simulink model "Minh_Final_project_Inverter_V3"  (R2024b)
settings: Solver=VariableStepAuto  StartTime=0.0  StopTime=100  FixedStep=1e-5  MaxStep=1e-3  MinStep=1e-8  RelTol=1e-2
values from neighbouring files (symbols this model uses):
  A_f = 1.24    [Minh_Inverter_Init.m]
  C_d = 0.7041    [Minh_Inverter_Init.m]
  C_rr = 0.02    [Minh_Inverter_Init.m]
  Current_max = min(InvCurr,mCurr)    [Minh_Inverter_Init.m]
  Encoder_Offset = (PhaseA_offset/ppair)*pi/180    (= -0.785398163397)    [Minh_Inverter_Init.m]
  g = 9.8    [Minh_Inverter_Init.m]
  J = mrot*r^2/k^2 + 0.0045    (= 0.8303048)    [Minh_Inverter_Init.m]
  k = 1    [Minh_Inverter_Init.m]
  lambda = 0.0375    [Minh_Inverter_Init.m]
  Ld = 0.1e-3    (= 0.0001)    [Minh_Inverter_Init.m]
  Lq = Ld    (= 0.0001)    [Minh_Inverter_Init.m]
  m = 1    [Minh_Inverter_Init.m]
  ppair = 4    [Minh_Inverter_Init.m]
  r = 0.4064/2    (= 0.2032)    [Minh_Inverter_Init.m]
  rho = 1.2    [Minh_Inverter_Init.m]
  Rs = (Rpp^2)/(Rpp*3)    (= 0.00433333333333)    [Minh_Inverter_Init.m]
  speed_max = rpm_max*2*pi/60    (= 523.598775598)    [Minh_Inverter_Init.m]
  Torque_max = Current_max*3*lambda*ppair/2    [Minh_Inverter_Init.m]
  Voltage_max = min(V_bat,mVolt)    [Minh_Inverter_Init.m]
undefined symbols (not defined in the file or in its folder): Down, Up
libraries: nesl_utility x27, fl_lib x23, slpidlib x12, ee_lib x11, spsabctodq0Lib x4, simulink x3, spsdq0toabcLib x2, eePwmGenerator x2, mcbresolverdecoderlib x1, eeResolverToDigitalConverter x1
(part 1 of 3)
settings Model: ExtModeTrigDuration=8  Creator=minhp  LastModifiedBy=minhp
settings SolverCC: ZeroCrossControl=DisableAll  ZeroCrossAlgorithm=Adaptive
settings OptimizationCC: DefaultParameterBehavior=Inlined  UseDivisionForNetSlopeComputation=on  GainParamInheritBuiltInType=on  UseFloatMulNetSlope=on  DefaultUnderspecifiedDataType=single  InlineInvariantSignals=on  PassReuseOutputArgsAs=Individual arguments  ZeroExternalMemoryAtStartup=off  NoFixptDivByZeroProtection=on  EfficientFloat2IntCast=on  LifeSpan=1  MaxStackSize=1024  OptimizeBlockOrder=speed  DifferentSizesBufferReuse=on  EfficientTunableParamExpr=on
settings DebuggingCC: MaskedZcDiagnostic=none  IgnoredZcDiagnostic=none  ParameterTunabilityLossMsg=error
settings HardwareCC: ProdBitPerChar=16  ProdBitPerInt=16  ProdBitPerPointer=32  ProdBitPerSizeT=32  ProdBitPerPtrDiffT=32  ProdLargestAtomicInteger=Integer  ProdLargestAtomicFloat=None  ProdWordSize=16  ProdLongLongMode=on  ProdHWDeviceType=Texas Instruments->C2000  HardwareBoardFeatureSet=SoCBlockset
settings SFSimCC: MATLABDynamicMemAlloc=off
settings RTWCC: Description=Embedded Coder  SystemTargetFile=ert.tlc  HardwareBoard=TI Piccolo F280049C LaunchPad  GenCodeOnly=on  TemplateMakefile=ert_default_tmf  Toolchain=Texas Instruments Code Composer Studio (C2000)  CodeProfilingSaveOptions=MetricsOnly
settings CodeAppCC: ForceParamTrailComments=on  IgnoreCustomStorageClasses=off  OperatorAnnotations=on  SimulinkDataObjDesc=on  SFDataObjDesc=on  CustomSymbolStrGlobalVar=rt$N$M  CustomSymbolStrType=$N$M  CustomSymbolStrFcn=$N$M$F  CustomSymbolStrMacro=$N$M  InsertBlockDesc=on
settings ERTTargetCC: CodeReplacementLibrary=TI C28x  IncludeMdlTerminateFcn=off  CombineSignalStateStructs=on  SupportAbsoluteTime=off  SupportComplex=off  SupportContinuousTime=on  ExtModeTransport=4  ExtModeStaticAlloc=on  ExtModeAutomaticAllocSize=off  ExtModeStaticAllocSize=5000  ExtModeMexFile=ext_xcp  ExtModeIntrfLevel=Level2 - Open  ERTFilePackagingFormat=CompactWithDataFile  DynamicArrayContainerType=coder::array

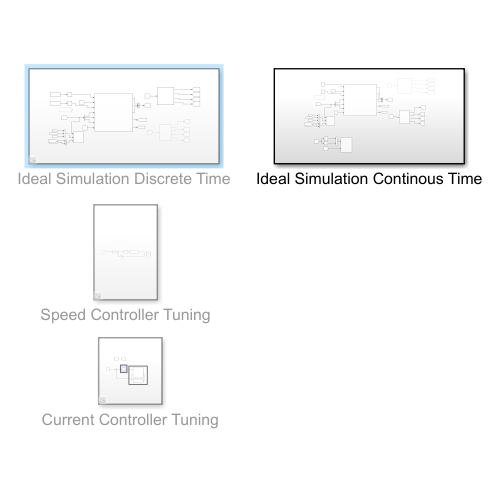
[thumbnail: Simulink's stored preview of the top-level diagram]
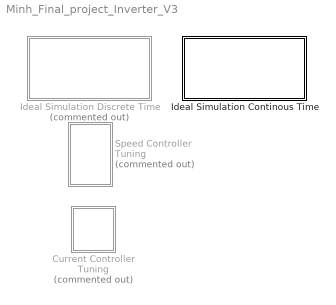
== system Minh_Final_project_Inverter_V3 ==
  Current Controller Tuning : Subsystem  Commented=on
  Ideal Simulation Continous Time : Subsystem
  Ideal Simulation Discrete Time : Subsystem  Commented=on
  Speed Controller Tuning : Subsystem  Commented=on

== system Minh_Final_project_Inverter_V3/Current Controller Tuning ==
  note: Use the PID tuner app to tune for bandwidth of at least 2000rad/s
      | and PM of 90deg
  note: Q current
      | Cntrl
  note: PMSM (Mathematical Model)
  I_dq PID : slpidlib/PID Controller  Controller=PI  Form=Parallel  TimeDomain=Continuous-time  UseExternalTs=off  SampleTime=-1  IntegratorMethod=Forward Euler  FilterMethod=Forward Euler  ControllerParametersSource=internal  P=0.199995991549269  I=7.0005743607815  UseKiTs=off  D=2.81416629288768e-05  UseExternalDerivativeSource=off  N=4271.19819316481  UseFilter=on  TunerSelectOption=Transfer Function Based (PID Tuner App)  InitialConditionSource=internal  InitialConditionForIntegrator=0  InitialConditionForFilter=0  DifferentiatorICPrevScaledInput=0  ExternalReset=none  TrackingMode=off  Kt=1  LimitOutput=on  SatLimitsSource=internal  UpperSaturationLimit=Voltage_max  LowerSaturationLimit=-Voltage_max  LinearizeAsGain=off  AntiWindupMode=none  Kb=1  LimitIntegrator=on  UpperIntegratorSaturationLimit=Voltage_max  LowerIntegratorSaturationLimit=-Voltage_max  POutMin=[]  POutMax=[]  IOutMin=[]  IOutMax=[]  DOutMin=[]  DOutMax=[]  NOutMin=[]  NOutMax=[]  SumOutMin=[]  SumOutMax=[]  SaturationOutMin=[]  SaturationOutMax=[]  PParamMin=[]  PParamMax=[]  IParamMin=[]  IParamMax=[]  DParamMin=[]  DParamMax=[]  NParamMin=[]  NParamMax=[]  KbParamMin=[]  KbParamMax=[]  KtParamMin=[]  KtParamMax=[]  KbOutMin=[]  KbOutMax=[]  KtOutMin=[]  KtOutMax=[]  IntegratorOutMin=[]  IntegratorOutMax=[]  FilterOutMin=[]  FilterOutMax=[]  SumI1OutMin=[]  SumI1OutMax=[]  SumI2OutMin=[]  SumI2OutMax=[]  SumI3OutMin=[]  SumI3OutMax=[]  SumI4OutMin=[]  SumI4OutMax=[]  SumDOutMin=[]  SumDOutMax=[]  DifferentiatorOutMin=[]  DifferentiatorOutMax=[]  FilterDiffOutCoefMin=[]  FilterDiffOutCoefMax=[]  ReciprocalOutMin=[]  ReciprocalOutMax=[]  SumDenOutMin=[]  SumDenOutMax=[]  SumNumOutMin=[]  SumNumOutMax=[]  DivideOutMin=[]  DivideOutMax=[]  UdiffTsProdOutMin=[]  UdiffTsProdOutMax=[]  NTsProdOutMin=[]  NTsProdOutMax=[]  UintegralTsProdOutMin=[]  UintegralTsProdOutMax=[]  UngainTsProdOutMin=[]  UngainTsProdOutMax=[]  ClampingZeroOutDataTypeStr=Inherit: Inherit via back propagation  ClampingZeroOutMin=[]  ClampingZeroOutMax=[]  FilterDenConstantOutDataTypeStr=Inherit: Inherit via back propagation  FilterDenConstantOutMin=[]  FilterDenConstantOutMax=[]  PCopyOutDataTypeStr=Inherit: Inherit via back propagation  PCopyOutMin=[]  PCopyOutMax=[]  NCopyOutDataTypeStr=Inherit: Inherit via back propagation  NCopyOutMin=[]  NCopyOutMax=[]  IntegratorContinuousStateAttributes=''  IntegratorStateMustResolveToSignalObject=off  IntegratorRTWStateStorageClass=Auto  FilterContinuousStateAttributes=''  FilterStateMustResolveToSignalObject=off  FilterRTWStateStorageClass=Auto  ParallelPVariant=InternalParameters  IdealPVariant=Disabled  IVariant=InternalParameters  DVariant=Disabled  IntegratorVariant=Continuous  SatVariant=Enabled  AWVariant=Passthrough  PCopyVariant=Disabled  TRVariant=Disabled  FdbkBlocksVariant=Forward  IdealPFdbkVariant=Disabled  SatFdbkVariant=Disabled  DerivativeFilterVariant=Disabled  NVariant=Disabled  NCopyVariant=Disabled_SignalSpec  FilterICVariant=Disabled  IntegratorICVariant=InternalICs  ExternalResetVariant=Disabled  TRSumVariant=Passthrough  SumFdbkVariant=Disabled  SumVariant=Sum_PI  TsampFilterVariant=InternalTs  TsampNgainVariant=Passthrough  TsampIntegralVariant=Disabled_SignalSpec  ExternalSaturationOutDataTypeStr=Inherit: Same as second input  DerivativeSourceVariant=Disabled  PreIntVariant=InternalPreInt
  I_dq PID1 : slpidlib/PID Controller  Commented=on  Controller=PID  Form=Parallel  TimeDomain=Discrete-time  UseExternalTs=off  SampleTime=-1  IntegratorMethod=Forward Euler  FilterMethod=Forward Euler  ControllerParametersSource=internal  P=0.183534072898089  I=62.295633089485  UseKiTs=off  D=2.81416629288768e-05  UseExternalDerivativeSource=off  N=4271.19819316481  UseFilter=on  TunerSelectOption=Transfer Function Based (PID Tuner App)  InitialConditionSource=internal  InitialConditionForIntegrator=0  InitialConditionForFilter=0  DifferentiatorICPrevScaledInput=0  ExternalReset=none  TrackingMode=off  Kt=1  LimitOutput=on  SatLimitsSource=internal  UpperSaturationLimit=Voltage_max  LowerSaturationLimit=-Voltage_max  LinearizeAsGain=off  AntiWindupMode=none  Kb=1  LimitIntegrator=on  UpperIntegratorSaturationLimit=Voltage_max  LowerIntegratorSaturationLimit=-Voltage_max  POutMin=[]  POutMax=[]  IOutMin=[]  IOutMax=[]  DOutMin=[]  DOutMax=[]  NOutMin=[]  NOutMax=[]  SumOutMin=[]  SumOutMax=[]  SaturationOutMin=[]  SaturationOutMax=[]  PParamMin=[]  PParamMax=[]  IParamMin=[]  IParamMax=[]  DParamMin=[]  DParamMax=[]  NParamMin=[]  NParamMax=[]  KbParamMin=[]  KbParamMax=[]  KtParamMin=[]  KtParamMax=[]  KbOutMin=[]  KbOutMax=[]  KtOutMin=[]  KtOutMax=[]  IntegratorOutMin=[]  IntegratorOutMax=[]  FilterOutMin=[]  FilterOutMax=[]  SumI1OutMin=[]  SumI1OutMax=[]  SumI2OutMin=[]  SumI2OutMax=[]  SumI3OutMin=[]  SumI3OutMax=[]  SumI4OutMin=[]  SumI4OutMax=[]  SumDOutMin=[]  SumDOutMax=[]  DifferentiatorOutMin=[]  DifferentiatorOutMax=[]  FilterDiffOutCoefMin=[]  FilterDiffOutCoefMax=[]  ReciprocalOutMin=[]  ReciprocalOutMax=[]  SumDenOutMin=[]  SumDenOutMax=[]  SumNumOutMin=[]  SumNumOutMax=[]  DivideOutMin=[]  DivideOutMax=[]  UdiffTsProdOutMin=[]  UdiffTsProdOutMax=[]  NTsProdOutMin=[]  NTsProdOutMax=[]  UintegralTsProdOutMin=[]  UintegralTsProdOutMax=[]  UngainTsProdOutMin=[]  UngainTsProdOutMax=[]  ClampingZeroOutDataTypeStr=Inherit: Inherit via back propagation  ClampingZeroOutMin=[]  ClampingZeroOutMax=[]  FilterDenConstantOutDataTypeStr=Inherit: Inherit via back propagation  FilterDenConstantOutMin=[]  FilterDenConstantOutMax=[]  PCopyOutDataTypeStr=Inherit: Inherit via back propagation  PCopyOutMin=[]  PCopyOutMax=[]  NCopyOutDataTypeStr=Inherit: Inherit via back propagation  NCopyOutMin=[]  NCopyOutMax=[]  IntegratorContinuousStateAttributes=''  IntegratorStateMustResolveToSignalObject=off  IntegratorRTWStateStorageClass=Auto  FilterContinuousStateAttributes=''  FilterStateMustResolveToSignalObject=off  FilterRTWStateStorageClass=Auto  ParallelPVariant=InternalParameters  IdealPVariant=Disabled  IVariant=InternalParameters  DVariant=InternalParameters  IntegratorVariant=Discrete  SatVariant=Enabled  AWVariant=Passthrough  PCopyVariant=Disabled  TRVariant=Disabled  FdbkBlocksVariant=Forward  IdealPFdbkVariant=Disabled  SatFdbkVariant=Disabled  DerivativeFilterVariant=ForwardEulerFilter  NVariant=InternalParameters  NCopyVariant=Disabled  FilterICVariant=InternalICsFilter  IntegratorICVariant=InternalICs  ExternalResetVariant=Disabled  TRSumVariant=Passthrough  SumFdbkVariant=Disabled  SumVariant=Sum_PID  TsampFilterVariant=InternalTs  TsampNgainVariant=Passthrough  TsampIntegralVariant=Disabled_SignalSpec  ExternalSaturationOutDataTypeStr=Inherit: Same as second input  DerivativeSourceVariant=ErrorSignal  PreIntVariant=InternalPreInt
  I_dq PID2 : slpidlib/PID Controller  Commented=on  Controller=PI  Form=Parallel  TimeDomain=Discrete-time  UseExternalTs=off  SampleTime=-1  IntegratorMethod=Forward Euler  FilterMethod=Forward Euler  ControllerParametersSource=internal  P=0.216674080570424  I=8.23559930371868  UseKiTs=off  D=2.81416629288768e-05  UseExternalDerivativeSource=off  N=4271.19819316481  UseFilter=on  TunerSelectOption=Transfer Function Based (PID Tuner App)  InitialConditionSource=internal  InitialConditionForIntegrator=0  InitialConditionForFilter=0  DifferentiatorICPrevScaledInput=0  ExternalReset=none  TrackingMode=off  Kt=1  LimitOutput=on  SatLimitsSource=internal  UpperSaturationLimit=Voltage_max  LowerSaturationLimit=-Voltage_max  LinearizeAsGain=off  AntiWindupMode=none  Kb=1  LimitIntegrator=on  UpperIntegratorSaturationLimit=Voltage_max  LowerIntegratorSaturationLimit=-Voltage_max  POutMin=[]  POutMax=[]  IOutMin=[]  IOutMax=[]  DOutMin=[]  DOutMax=[]  NOutMin=[]  NOutMax=[]  SumOutMin=[]  SumOutMax=[]  SaturationOutMin=[]  SaturationOutMax=[]  PParamMin=[]  PParamMax=[]  IParamMin=[]  IParamMax=[]  DParamMin=[]  DParamMax=[]  NParamMin=[]  NParamMax=[]  KbParamMin=[]  KbParamMax=[]  KtParamMin=[]  KtParamMax=[]  KbOutMin=[]  KbOutMax=[]  KtOutMin=[]  KtOutMax=[]  IntegratorOutMin=[]  IntegratorOutMax=[]  FilterOutMin=[]  FilterOutMax=[]  SumI1OutMin=[]  SumI1OutMax=[]  SumI2OutMin=[]  SumI2OutMax=[]  SumI3OutMin=[]  SumI3OutMax=[]  SumI4OutMin=[]  SumI4OutMax=[]  SumDOutMin=[]  SumDOutMax=[]  DifferentiatorOutMin=[]  DifferentiatorOutMax=[]  FilterDiffOutCoefMin=[]  FilterDiffOutCoefMax=[]  ReciprocalOutMin=[]  ReciprocalOutMax=[]  SumDenOutMin=[]  SumDenOutMax=[]  SumNumOutMin=[]  SumNumOutMax=[]  DivideOutMin=[]  DivideOutMax=[]  UdiffTsProdOutMin=[]  UdiffTsProdOutMax=[]  NTsProdOutMin=[]  NTsProdOutMax=[]  UintegralTsProdOutMin=[]  UintegralTsProdOutMax=[]  UngainTsProdOutMin=[]  UngainTsProdOutMax=[]  ClampingZeroOutDataTypeStr=Inherit: Inherit via back propagation  ClampingZeroOutMin=[]  ClampingZeroOutMax=[]  FilterDenConstantOutDataTypeStr=Inherit: Inherit via back propagation  FilterDenConstantOutMin=[]  FilterDenConstantOutMax=[]  PCopyOutDataTypeStr=Inherit: Inherit via back propagation  PCopyOutMin=[]  PCopyOutMax=[]  NCopyOutDataTypeStr=Inherit: Inherit via back propagation  NCopyOutMin=[]  NCopyOutMax=[]  IntegratorContinuousStateAttributes=''  IntegratorStateMustResolveToSignalObject=off  IntegratorRTWStateStorageClass=Auto  FilterContinuousStateAttributes=''  FilterStateMustResolveToSignalObject=off  FilterRTWStateStorageClass=Auto  ParallelPVariant=InternalParameters  IdealPVariant=Disabled  IVariant=InternalParameters  DVariant=Disabled  IntegratorVariant=Discrete  SatVariant=Enabled  AWVariant=Passthrough  PCopyVariant=Disabled  TRVariant=Disabled  FdbkBlocksVariant=Forward  IdealPFdbkVariant=Disabled  SatFdbkVariant=Disabled  DerivativeFilterVariant=Disabled  NVariant=Disabled  NCopyVariant=Disabled_SignalSpec  FilterICVariant=Disabled  IntegratorICVariant=InternalICs  ExternalResetVariant=Disabled  TRSumVariant=Passthrough  SumFdbkVariant=Disabled  SumVariant=Sum_PI  TsampFilterVariant=InternalTs  TsampNgainVariant=Passthrough  TsampIntegralVariant=Disabled_SignalSpec  ExternalSaturationOutDataTypeStr=Inherit: Same as second input  DerivativeSourceVariant=Disabled  PreIntVariant=InternalPreInt
  Machine Model in DQ1 : Subsystem
  Mechanical Model : Subsystem
  Sum3 : Sum  Inputs=|+-
  current request1 : Constant  Value=10
  wires:
  Machine Model in DQ1/1(i_q) -> Sum3/2  "i_q"
  Machine Model in DQ1/2(T_e) -> Mechanical Model/1(T_e)  "Tourqe"
  current request1/1 -> Sum3/1
  Sum3/1 -> I_dq PID/1  "Iq_error"
  I_dq PID/1 -> Machine Model in DQ1/1(v_q)  "Vq*"
  Mechanical Model/1(w_m) -> Machine Model in DQ1/2(w_m)

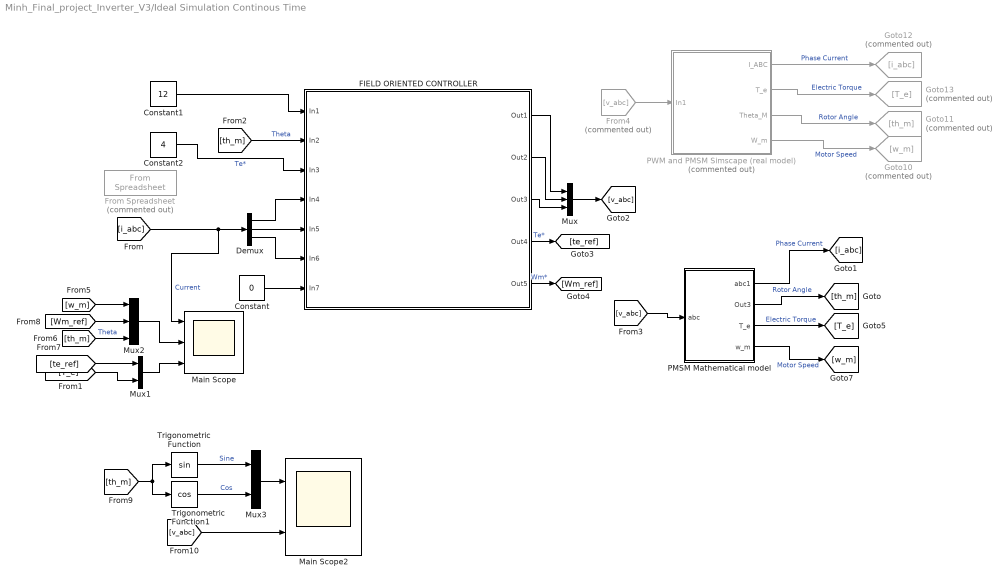
== system Minh_Final_project_Inverter_V3/Ideal Simulation Continous Time ==
  Constant : Constant  Value=0
  Constant1 : Constant  Value=12
  Constant2 : Constant  Value=4
  Demux : Demux  Outputs=3
  FIELD ORIENTED CONTROLLER : Subsystem
  From Spreadsheet : FromSpreadsheet  Commented=on  FileName=Inverter_Lap_Sim_Current_Calcs.xlsx
  From4 : From  Commented=on  GotoTag=v_abc
  Goto10 : Goto  Commented=on  GotoTag=w_m
  Goto11 : Goto  Commented=on  GotoTag=th_m
  Goto12 : Goto  Commented=on  GotoTag=i_abc
  Goto13 : Goto  Commented=on  GotoTag=T_e
  Main Scope : Scope  NumInputPorts=3
  Main Scope2 : Scope  NumInputPorts=2
  Mux : Mux  Inputs=3
  Mux1 : Mux  Inputs=2
  Mux2 : Mux  Inputs=3
  Mux3 : Mux  Inputs=2
  PMSM Mathematical model : Subsystem
  PWM and PMSM Simscape (real model) : Subsystem  Commented=on
  Trigonometric Function : Trigonometry
  Trigonometric Function1 : Trigonometry  Operator=cos
  wires:
  [th_m] -> FIELD ORIENTED CONTROLLER/2(In2)  "Theta"
  FIELD ORIENTED CONTROLLER/3(Out3) -> Mux/3
  [i_abc] -> Main Scope/1, Demux/1  "Current"
  Mux2/1 -> Main Scope/2
  [te_ref] -> Mux1/1
  Constant/1 -> FIELD ORIENTED CONTROLLER/7(In7)
  PWM and PMSM Simscape (real model)/3(Theta_M) -> Goto11/1  "Rotor Angle"
  [T_e] -> Mux1/2
  FIELD ORIENTED CONTROLLER/2(Out2) -> Mux/2
  Demux/3 -> FIELD ORIENTED CONTROLLER/6(In6)
  FIELD ORIENTED CONTROLLER/5(Out5) -> [Wm_ref]  "Wm*"
  Demux/2 -> FIELD ORIENTED CONTROLLER/5(In5)
  PMSM Mathematical model/4(w_m) -> [w_m]  "Motor Speed"
  FIELD ORIENTED CONTROLLER/4(Out4) -> [te_ref]  "Te*"
  FIELD ORIENTED CONTROLLER/1(Out1) -> Mux/1
  PMSM Mathematical model/2(Out3) -> [th_m]  "Rotor Angle"
  Demux/1 -> FIELD ORIENTED CONTROLLER/4(In4)
  Mux/1 -> [v_abc]
  [th_m] -> Mux2/3  "Theta"
  [w_m] -> Mux2/1
  PWM and PMSM Simscape (real model)/2(T_e) -> Goto13/1  "Electric Torque"
  Constant2/1 -> FIELD ORIENTED CONTROLLER/3(In3)  "Te*"
  PWM and PMSM Simscape (real model)/1(I_ABC) -> Goto12/1  "Phase Current"
  From4/1 -> PWM and PMSM Simscape (real model)/1(In1)
  PWM and PMSM Simscape (real model)/4(W_m) -> Goto10/1  "Motor Speed"
  [v_abc] -> PMSM Mathematical model/1(abc)
  PMSM Mathematical model/1(abc1) -> [i_abc]  "Phase Current"
  PMSM Mathematical model/3(T_e) -> [T_e]  "Electric Torque"
  Constant1/1 -> FIELD ORIENTED CONTROLLER/1(In1)
  [Wm_ref] -> Mux2/2
  Mux1/1 -> Main Scope/3
  Trigonometric Function1/1 -> Mux3/2  "Cos"
  Mux3/1 -> Main Scope2/1
  [v_abc] -> Main Scope2/2
  Trigonometric Function/1 -> Mux3/1  "Sine"
  [th_m] -> Trigonometric Function1/1, Trigonometric Function/1

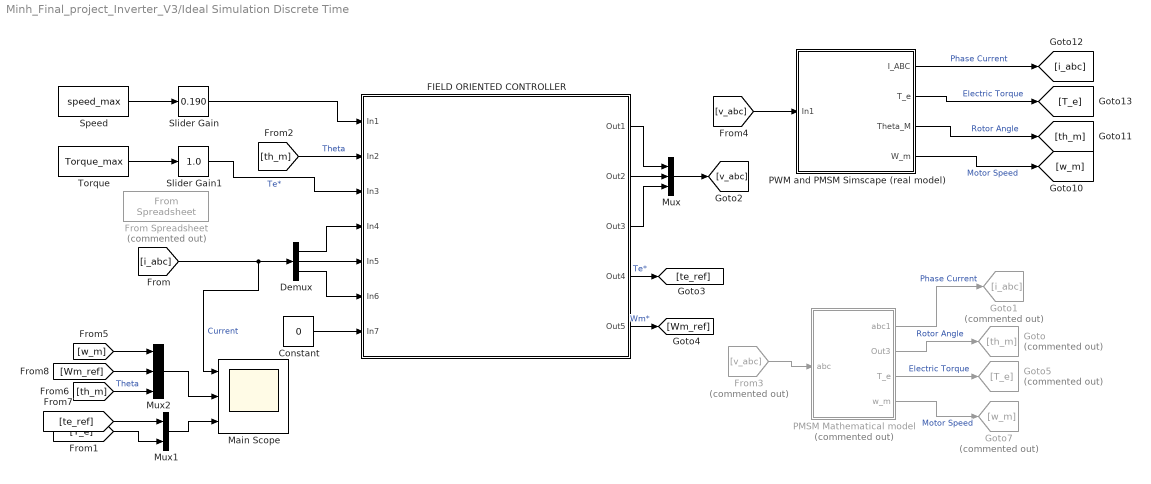
== system Minh_Final_project_Inverter_V3/Ideal Simulation Discrete Time ==
  Constant : Constant  Value=0
  Demux : Demux  Outputs=3
  FIELD ORIENTED CONTROLLER : Subsystem
  From Spreadsheet : FromSpreadsheet  Commented=on  FileName=Inverter_Lap_Sim_Current_Calcs.xlsx
  From3 : From  Commented=on  GotoTag=v_abc
  Goto : Goto  Commented=on  GotoTag=th_m
  Goto1 : Goto  Commented=on  GotoTag=i_abc
  Goto5 : Goto  Commented=on  GotoTag=T_e
  Goto7 : Goto  Commented=on  GotoTag=w_m
  Main Scope : Scope  NumInputPorts=3
  Mux : Mux  Inputs=3
  Mux1 : Mux  Inputs=2
  Mux2 : Mux  Inputs=3
  PMSM Mathematical model : Subsystem  Commented=on
  PWM and PMSM Simscape (real model) : Subsystem
  Slider Gain : simulink/Math Operations/Slider Gain  gain=0.190  low=0  high=1
  Slider Gain1 : simulink/Math Operations/Slider Gain  gain=1.0  low=0  high=1
  Speed : Constant  Value=speed_max
  Torque : Constant  Value=Torque_max
  wires:
  [th_m] -> FIELD ORIENTED CONTROLLER/2(In2)  "Theta"
  FIELD ORIENTED CONTROLLER/3(Out3) -> Mux/3
  [i_abc] -> Main Scope/1, Demux/1  "Current"
  Mux2/1 -> Main Scope/2
  [te_ref] -> Mux1/1
  Constant/1 -> FIELD ORIENTED CONTROLLER/7(In7)
  PWM and PMSM Simscape (real model)/3(Theta_M) -> [th_m]  "Rotor Angle"
  [T_e] -> Mux1/2
  FIELD ORIENTED CONTROLLER/2(Out2) -> Mux/2
  Demux/3 -> FIELD ORIENTED CONTROLLER/6(In6)
  FIELD ORIENTED CONTROLLER/5(Out5) -> [Wm_ref]  "Wm*"
  Torque/1 -> Slider Gain1/1
  Demux/2 -> FIELD ORIENTED CONTROLLER/5(In5)
  PMSM Mathematical model/4(w_m) -> Goto7/1  "Motor Speed"
  FIELD ORIENTED CONTROLLER/4(Out4) -> [te_ref]  "Te*"
  FIELD ORIENTED CONTROLLER/1(Out1) -> Mux/1
  PMSM Mathematical model/2(Out3) -> Goto/1  "Rotor Angle"
  Demux/1 -> FIELD ORIENTED CONTROLLER/4(In4)
  Mux/1 -> [v_abc]
  [th_m] -> Mux2/3  "Theta"
  [w_m] -> Mux2/1
  PWM and PMSM Simscape (real model)/2(T_e) -> [T_e]  "Electric Torque"
  Slider Gain1/1 -> FIELD ORIENTED CONTROLLER/3(In3)  "Te*"
  PWM and PMSM Simscape (real model)/1(I_ABC) -> [i_abc]  "Phase Current"
  [v_abc] -> PWM and PMSM Simscape (real model)/1(In1)
  PWM and PMSM Simscape (real model)/4(W_m) -> [w_m]  "Motor Speed"
  From3/1 -> PMSM Mathematical model/1(abc)
  PMSM Mathematical model/1(abc1) -> Goto1/1  "Phase Current"
  PMSM Mathematical model/3(T_e) -> Goto5/1  "Electric Torque"
  Slider Gain/1 -> FIELD ORIENTED CONTROLLER/1(In1)
  [Wm_ref] -> Mux2/2
  Speed/1 -> Slider Gain/1
  Mux1/1 -> Main Scope/3

== system Minh_Final_project_Inverter_V3/Speed Controller Tuning ==
  note: Tuned for 100rad/s BW and 90deg PM
  Gain2 : Gain  Gain=ppair
  Gain7 : Gain  Gain=ppair
  Mechanical Model : Subsystem
  Speed PID : slpidlib/PID Controller  Commented=on  Controller=PD  Form=Parallel  TimeDomain=Discrete-time  UseExternalTs=off  SampleTime=-1  IntegratorMethod=Forward Euler  FilterMethod=Forward Euler  ControllerParametersSource=internal  P=20.6545195236646  I=640.266262711417  UseKiTs=off  D=0.00205517598679868  UseExternalDerivativeSource=off  N=100.498329175013  UseFilter=on  TunerSelectOption=Transfer Function Based (PID Tuner App)  InitialConditionSource=internal  InitialConditionForIntegrator=0  InitialConditionForFilter=0  DifferentiatorICPrevScaledInput=0  ExternalReset=none  TrackingMode=off  Kt=1  LimitOutput=on  SatLimitsSource=internal  UpperSaturationLimit=Torque_max  LowerSaturationLimit=-Torque_max  LinearizeAsGain=off  AntiWindupMode=none  Kb=1  LimitIntegrator=on  UpperIntegratorSaturationLimit=Torque_max  LowerIntegratorSaturationLimit=-Torque_max  RndMeth=Nearest  POutMin=[]  POutMax=[]  IOutMin=[]  IOutMax=[]  DOutMin=[]  DOutMax=[]  NOutMin=[]  NOutMax=[]  SumOutMin=[]  SumOutMax=[]  SaturationOutMin=[]  SaturationOutMax=[]  PParamMin=[]  PParamMax=[]  IParamMin=[]  IParamMax=[]  DParamMin=[]  DParamMax=[]  NParamMin=[]  NParamMax=[]  KbParamMin=[]  KbParamMax=[]  KtParamMin=[]  KtParamMax=[]  KbOutMin=[]  KbOutMax=[]  KtOutMin=[]  KtOutMax=[]  IntegratorOutMin=[]  IntegratorOutMax=[]  FilterOutMin=[]  FilterOutMax=[]  SumI1OutMin=[]  SumI1OutMax=[]  SumI2OutMin=[]  SumI2OutMax=[]  SumI3OutMin=[]  SumI3OutMax=[]  SumI4OutMin=[]  SumI4OutMax=[]  SumDOutMin=[]  SumDOutMax=[]  DifferentiatorOutMin=[]  DifferentiatorOutMax=[]  FilterDiffOutCoefMin=[]  FilterDiffOutCoefMax=[]  ReciprocalOutMin=[]  ReciprocalOutMax=[]  SumDenOutMin=[]  SumDenOutMax=[]  SumNumOutMin=[]  SumNumOutMax=[]  DivideOutMin=[]  DivideOutMax=[]  UdiffTsProdOutMin=[]  UdiffTsProdOutMax=[]  NTsProdOutMin=[]  NTsProdOutMax=[]  UintegralTsProdOutMin=[]  UintegralTsProdOutMax=[]  UngainTsProdOutMin=[]  UngainTsProdOutMax=[]  ClampingZeroOutDataTypeStr=Inherit: Inherit via back propagation  ClampingZeroOutMin=[]  ClampingZeroOutMax=[]  FilterDenConstantOutDataTypeStr=Inherit: Inherit via back propagation  FilterDenConstantOutMin=[]  FilterDenConstantOutMax=[]  PCopyOutDataTypeStr=Inherit: Inherit via back propagation  PCopyOutMin=[]  PCopyOutMax=[]  NCopyOutDataTypeStr=Inherit: Inherit via back propagation  NCopyOutMin=[]  NCopyOutMax=[]  IntegratorContinuousStateAttributes=''  IntegratorStateMustResolveToSignalObject=off  IntegratorRTWStateStorageClass=Auto  FilterContinuousStateAttributes=''  FilterStateMustResolveToSignalObject=off  FilterRTWStateStorageClass=Auto  ParallelPVariant=InternalParameters  IdealPVariant=Disabled  IVariant=Disabled  DVariant=InternalParameters  IntegratorVariant=Disabled  SatVariant=Enabled  AWVariant=Disabled  PCopyVariant=Disabled  TRVariant=Disabled  FdbkBlocksVariant=Forward  IdealPFdbkVariant=Disabled  SatFdbkVariant=Disabled  DerivativeFilterVariant=ForwardEulerFilter  NVariant=InternalParameters  NCopyVariant=Disabled  FilterICVariant=InternalICsFilter  IntegratorICVariant=Disabled  ExternalResetVariant=Disabled  TRSumVariant=Passthrough  SumFdbkVariant=Disabled  SumVariant=Sum_PD  TsampFilterVariant=InternalTs  TsampNgainVariant=Passthrough  TsampIntegralVariant=Disabled_SignalSpec  ExternalSaturationOutDataTypeStr=Inherit: Same as second input  DerivativeSourceVariant=ErrorSignal  PreIntVariant=InternalPreInt
  Speed PID1 : slpidlib/PID Controller  Commented=on  Controller=PID  Form=Parallel  TimeDomain=Discrete-time  UseExternalTs=off  SampleTime=-1  IntegratorMethod=Forward Euler  FilterMethod=Forward Euler  ControllerParametersSource=internal  P=72.5692906092283  I=640.266262711417  UseKiTs=off  D=0.279453610046526  UseExternalDerivativeSource=off  N=180.694180073373  UseFilter=on  TunerSelectOption=Transfer Function Based (PID Tuner App)  InitialConditionSource=internal  InitialConditionForIntegrator=0  InitialConditionForFilter=0  DifferentiatorICPrevScaledInput=0  ExternalReset=none  TrackingMode=off  Kt=1  LimitOutput=on  SatLimitsSource=internal  UpperSaturationLimit=Torque_max  LowerSaturationLimit=-Torque_max  LinearizeAsGain=off  AntiWindupMode=none  Kb=1  LimitIntegrator=on  UpperIntegratorSaturationLimit=Torque_max  LowerIntegratorSaturationLimit=-Torque_max  RndMeth=Nearest  POutMin=[]  POutMax=[]  IOutMin=[]  IOutMax=[]  DOutMin=[]  DOutMax=[]  NOutMin=[]  NOutMax=[]  SumOutMin=[]  SumOutMax=[]  SaturationOutMin=[]  SaturationOutMax=[]  PParamMin=[]  PParamMax=[]  IParamMin=[]  IParamMax=[]  DParamMin=[]  DParamMax=[]  NParamMin=[]  NParamMax=[]  KbParamMin=[]  KbParamMax=[]  KtParamMin=[]  KtParamMax=[]  KbOutMin=[]  KbOutMax=[]  KtOutMin=[]  KtOutMax=[]  IntegratorOutMin=[]  IntegratorOutMax=[]  FilterOutMin=[]  FilterOutMax=[]  SumI1OutMin=[]  SumI1OutMax=[]  SumI2OutMin=[]  SumI2OutMax=[]  SumI3OutMin=[]  SumI3OutMax=[]  SumI4OutMin=[]  SumI4OutMax=[]  SumDOutMin=[]  SumDOutMax=[]  DifferentiatorOutMin=[]  DifferentiatorOutMax=[]  FilterDiffOutCoefMin=[]  FilterDiffOutCoefMax=[]  ReciprocalOutMin=[]  ReciprocalOutMax=[]  SumDenOutMin=[]  SumDenOutMax=[]  SumNumOutMin=[]  SumNumOutMax=[]  DivideOutMin=[]  DivideOutMax=[]  UdiffTsProdOutMin=[]  UdiffTsProdOutMax=[]  NTsProdOutMin=[]  NTsProdOutMax=[]  UintegralTsProdOutMin=[]  UintegralTsProdOutMax=[]  UngainTsProdOutMin=[]  UngainTsProdOutMax=[]  ClampingZeroOutDataTypeStr=Inherit: Inherit via back propagation  ClampingZeroOutMin=[]  ClampingZeroOutMax=[]  FilterDenConstantOutDataTypeStr=Inherit: Inherit via back propagation  FilterDenConstantOutMin=[]  FilterDenConstantOutMax=[]  PCopyOutDataTypeStr=Inherit: Inherit via back propagation  PCopyOutMin=[]  PCopyOutMax=[]  NCopyOutDataTypeStr=Inherit: Inherit via back propagation  NCopyOutMin=[]  NCopyOutMax=[]  IntegratorContinuousStateAttributes=''  IntegratorStateMustResolveToSignalObject=off  IntegratorRTWStateStorageClass=Auto  FilterContinuousStateAttributes=''  FilterStateMustResolveToSignalObject=off  FilterRTWStateStorageClass=Auto  ParallelPVariant=InternalParameters  IdealPVariant=Disabled  IVariant=InternalParameters  DVariant=InternalParameters  IntegratorVariant=Discrete  SatVariant=Enabled  AWVariant=Passthrough  PCopyVariant=Disabled  TRVariant=Disabled  FdbkBlocksVariant=Forward  IdealPFdbkVariant=Disabled  SatFdbkVariant=Disabled  DerivativeFilterVariant=ForwardEulerFilter  NVariant=InternalParameters  NCopyVariant=Disabled  FilterICVariant=InternalICsFilter  IntegratorICVariant=InternalICs  ExternalResetVariant=Disabled  TRSumVariant=Passthrough  SumFdbkVariant=Disabled  SumVariant=Sum_PID  TsampFilterVariant=InternalTs  TsampNgainVariant=Passthrough  TsampIntegralVariant=Disabled_SignalSpec  ExternalSaturationOutDataTypeStr=Inherit: Same as second input  DerivativeSourceVariant=ErrorSignal  PreIntVariant=InternalPreInt
  Speed PID2 : slpidlib/PID Controller  Controller=PD  Form=Parallel  TimeDomain=Continuous-time  UseExternalTs=off  SampleTime=-1  IntegratorMethod=Forward Euler  FilterMethod=Forward Euler  ControllerParametersSource=internal  P=20.75762  I=640.266262711417  UseKiTs=off  D=0  UseExternalDerivativeSource=off  N=100  UseFilter=on  TunerSelectOption=Transfer Function Based (PID Tuner App)  InitialConditionSource=internal  InitialConditionForIntegrator=0  InitialConditionForFilter=0  DifferentiatorICPrevScaledInput=0  ExternalReset=none  TrackingMode=off  Kt=1  LimitOutput=on  SatLimitsSource=internal  UpperSaturationLimit=Torque_max  LowerSaturationLimit=-Torque_max  LinearizeAsGain=off  AntiWindupMode=none  Kb=1  LimitIntegrator=on  UpperIntegratorSaturationLimit=Torque_max  LowerIntegratorSaturationLimit=-Torque_max  RndMeth=Nearest  POutMin=[]  POutMax=[]  IOutMin=[]  IOutMax=[]  DOutMin=[]  DOutMax=[]  NOutMin=[]  NOutMax=[]  SumOutMin=[]  SumOutMax=[]  SaturationOutMin=[]  SaturationOutMax=[]  PParamMin=[]  PParamMax=[]  IParamMin=[]  IParamMax=[]  DParamMin=[]  DParamMax=[]  NParamMin=[]  NParamMax=[]  KbParamMin=[]  KbParamMax=[]  KtParamMin=[]  KtParamMax=[]  KbOutMin=[]  KbOutMax=[]  KtOutMin=[]  KtOutMax=[]  IntegratorOutMin=[]  IntegratorOutMax=[]  FilterOutMin=[]  FilterOutMax=[]  SumI1OutMin=[]  SumI1OutMax=[]  SumI2OutMin=[]  SumI2OutMax=[]  SumI3OutMin=[]  SumI3OutMax=[]  SumI4OutMin=[]  SumI4OutMax=[]  SumDOutMin=[]  SumDOutMax=[]  DifferentiatorOutMin=[]  DifferentiatorOutMax=[]  FilterDiffOutCoefMin=[]  FilterDiffOutCoefMax=[]  ReciprocalOutMin=[]  ReciprocalOutMax=[]  SumDenOutMin=[]  SumDenOutMax=[]  SumNumOutMin=[]  SumNumOutMax=[]  DivideOutMin=[]  DivideOutMax=[]  UdiffTsProdOutMin=[]  UdiffTsProdOutMax=[]  NTsProdOutMin=[]  NTsProdOutMax=[]  UintegralTsProdOutMin=[]  UintegralTsProdOutMax=[]  UngainTsProdOutMin=[]  UngainTsProdOutMax=[]  ClampingZeroOutDataTypeStr=Inherit: Inherit via back propagation  ClampingZeroOutMin=[]  ClampingZeroOutMax=[]  FilterDenConstantOutDataTypeStr=Inherit: Inherit via back propagation  FilterDenConstantOutMin=[]  FilterDenConstantOutMax=[]  PCopyOutDataTypeStr=Inherit: Inherit via back propagation  PCopyOutMin=[]  PCopyOutMax=[]  NCopyOutDataTypeStr=Inherit: Inherit via back propagation  NCopyOutMin=[]  NCopyOutMax=[]  IntegratorContinuousStateAttributes=''  IntegratorStateMustResolveToSignalObject=off  IntegratorRTWStateStorageClass=Auto  FilterContinuousStateAttributes=''  FilterStateMustResolveToSignalObject=off  FilterRTWStateStorageClass=Auto  ParallelPVariant=InternalParameters  IdealPVariant=Disabled  IVariant=Disabled  DVariant=InternalParameters  IntegratorVariant=Disabled  SatVariant=Enabled  AWVariant=Disabled  PCopyVariant=Disabled  TRVariant=Disabled  FdbkBlocksVariant=Forward  IdealPFdbkVariant=Disabled  SatFdbkVariant=Disabled  DerivativeFilterVariant=ContFilter  NVariant=InternalParameters  NCopyVariant=Disabled  FilterICVariant=InternalICsFilter  IntegratorICVariant=Disabled  ExternalResetVariant=Disabled  TRSumVariant=Passthrough  SumFdbkVariant=Disabled  SumVariant=Sum_PD  TsampFilterVariant=InternalTs  TsampNgainVariant=Passthrough  TsampIntegralVariant=Disabled_SignalSpec  ExternalSaturationOutDataTypeStr=Inherit: Same as second input  DerivativeSourceVariant=ErrorSignal  PreIntVariant=InternalPreInt
  Speed request (Rad/s)2 : Constant  Value=1000
  Sum6 : Sum  Inputs=|+-
  wires:
  Mechanical Model/1(w_m) -> Gain2/1  "Electrical speed"
  Speed PID2/1 -> Mechanical Model/1(T_e)  "Te"
  Gain7/1 -> Sum6/1  "We*"
  Sum6/1 -> Speed PID2/1  "speed_err"
  Speed request (Rad/s)2/1 -> Gain7/1  "User_Spd_Req"
  Gain2/1 -> Sum6/2  "Electrical speed"

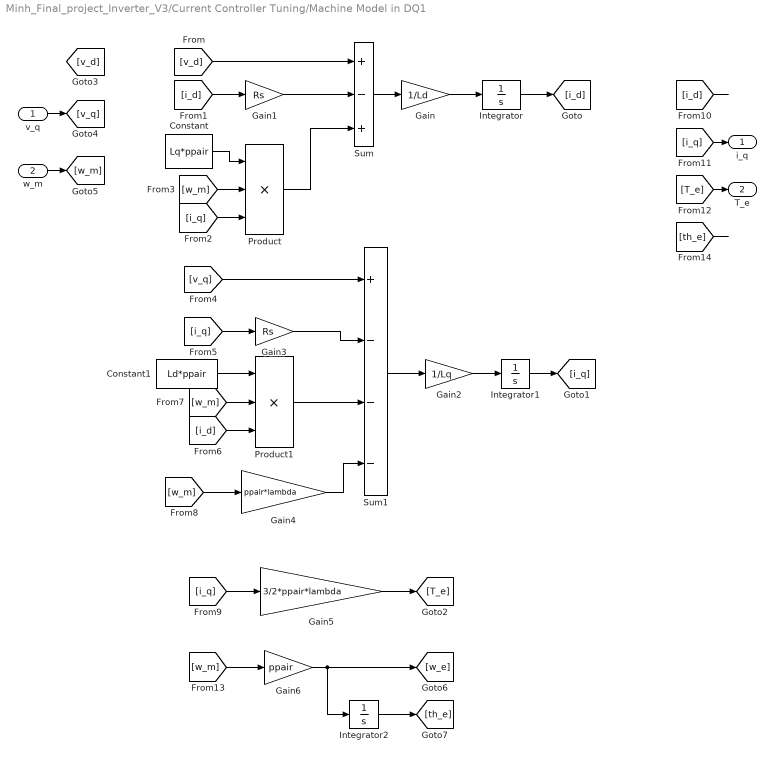
== system Minh_Final_project_Inverter_V3/Current Controller Tuning/Machine Model in DQ1 ==
  v_q : Inport
  w_m : Inport  Port=2
  Constant : Constant  Value=Lq*ppair
  Constant1 : Constant  Value=Ld*ppair
  Gain : Gain  Gain=1/Ld
  Gain1 : Gain  Gain=Rs
  Gain2 : Gain  Gain=1/Lq
  Gain3 : Gain  Gain=Rs
  Gain4 : Gain  Gain=ppair*lambda
  Gain5 : Gain  Gain=3/2*ppair*lambda
  Gain6 : Gain  Gain=ppair
  Integrator : Integrator
  Integrator1 : Integrator
  Integrator2 : Integrator
  Product : Product  Inputs=3
  Product1 : Product  Inputs=3
  Sum : Sum  Inputs=+-+
  Sum1 : Sum  Inputs=+---
  i_q : Outport
  T_e : Outport  Port=2
  wires:
  Constant/1 -> Product/1
  Product/1 -> Sum/3
  Integrator/1 -> [i_d]
  [v_d] -> Sum/1
  [w_m] -> Product1/2
  Gain4/1 -> Sum1/4
  [i_q] -> Product/3
  Sum/1 -> Gain/1
  [w_m] -> Gain4/1
  [i_d] -> Gain1/1
  Sum1/1 -> Gain2/1
  Gain/1 -> Integrator/1
  Gain5/1 -> [T_e]
  [i_q] -> Gain5/1
  Gain1/1 -> Sum/2
  Integrator1/1 -> [i_q]
  [i_q] -> Gain3/1
  Product1/1 -> Sum1/3
  Constant1/1 -> Product1/1
  Gain2/1 -> Integrator1/1
  [v_q] -> Sum1/1
  Gain3/1 -> Sum1/2
  [i_d] -> Product1/3
  [w_m] -> Product/2
  ? -> [v_d]
  v_q/1 -> [v_q]
  [i_d] -> ?
  [i_q] -> i_q/1
  [T_e] -> T_e/1
  w_m/1 -> [w_m]
  [w_m] -> Gain6/1
  Gain6/1 -> Integrator2/1, [w_e]
  Integrator2/1 -> [th_e]
  [th_e] -> ?

== system Minh_Final_project_Inverter_V3/Current Controller Tuning/Mechanical Model ==
  T_e : Inport
  Constant1 : Constant  Value=1/2*rho*C_d*A_f*r^2
  Gain : Gain  Gain=1/k^2
  Product2 : Product
  Square : Math  Operator=square
  Subtract : Sum  Inputs=|+-
  Transfer Fcn : TransferFcn  Denominator=[J 0]
  w_m : Outport
  wires:
  Constant1/1 -> Product2/1
  Transfer Fcn/1 -> Square/1, w_m/1
  Product2/1 -> Gain/1
  Square/1 -> Product2/2
  Subtract/1 -> Transfer Fcn/1
  T_e/1 -> Subtract/1
  Gain/1 -> Subtract/2

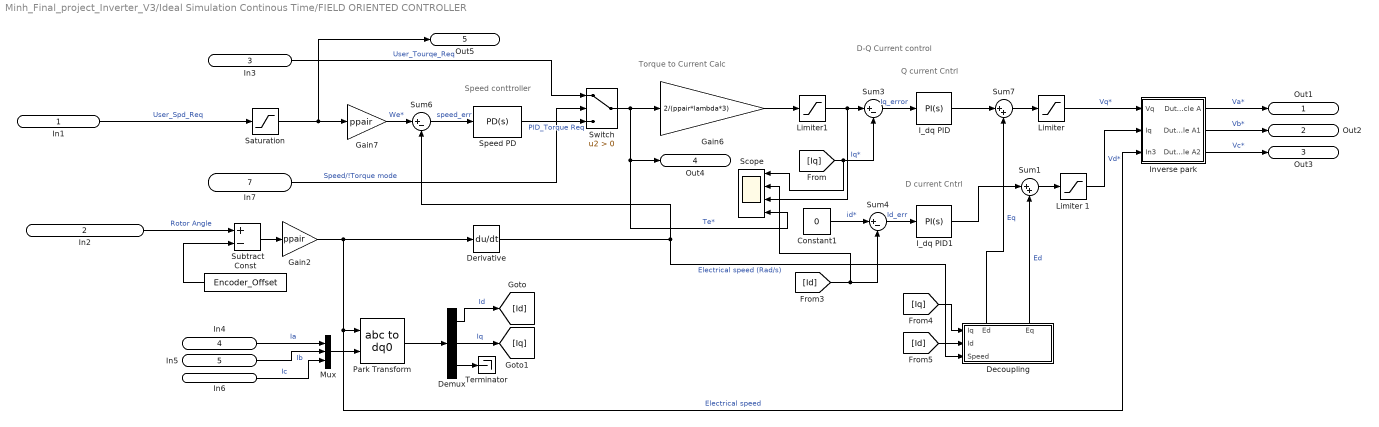
== system Minh_Final_project_Inverter_V3/Ideal Simulation Continous Time/FIELD ORIENTED CONTROLLER ==
  note: Torque to Current Calc
  note: Speed conttroller
  note: D current
      | Cntrl
  note: D-Q Current control
  note: Q current
      | Cntrl
  In1 : Inport
  In2 : Inport  Port=2
  In3 : Inport  Port=3
  In4 : Inport  Port=4
  In5 : Inport  Port=5
  In6 : Inport  Port=6
  In7 : Inport  Port=7
  Const : Constant  Value=Encoder_Offset
  Constant1 : Constant  Value=0
  Decoupling : Subsystem
      settings: PortSchema="{\"entries\":[{\"content\":{\"sides\":[{\"content\":{\"connectorIds\":[\"In1\",\"In2\",\"In3\"]},\"type\":\"ConnectorPlacement.EquallySpacedRectSide\",\"uuid\":\"5f512ccb-8595-4499-a419-e995908cd1f5\"},{\"content\":{\"side\":\"RIGHT\"},\"type\":\"ConnectorPlacement.EquallySpacedRectSide\",\"uuid\":\"2a1de219-597a-4818-9587-d28590d7f25d\"},{\"content\":{\"connectorIds\":[\"Out1\",\"Out2\"],\"side\":\"TOP\"},\"type\":\"ConnectorPlacement.EquallySpacedRectSide\",\"uuid\":\"87b053a8-3806-4156-bae7-a97f33c02d51\"}]},\"type\":\"ConnectorPlacement.EquallySpacedConnector\",\"uuid\":\"5d9f8914-d3c5-4fbe-94a4-f1d2e0d8a5f7\"}],\"packageUris\":[\"http://schema.mathworks.com/mf0/Connector/R2020b\"],\"version\":\"1.0\"}"
  Demux : Demux  Outputs=3
  Derivative : Derivative
  Gain2 : Gain  Gain=ppair
  Gain6 : Gain  Gain=2/(ppair*lambda*3)
  Gain7 : Gain  Gain=ppair
  I_dq PID : slpidlib/PID Controller  Controller=PI  Form=Parallel  TimeDomain=Continuous-time  UseExternalTs=off  SampleTime=-1  IntegratorMethod=Forward Euler  FilterMethod=Forward Euler  ControllerParametersSource=internal  P=0.199995991549269  I=7.0005743607815  UseKiTs=off  D=2.81416629288768e-05  UseExternalDerivativeSource=off  N=4271.19819316481  UseFilter=on  TunerSelectOption=Transfer Function Based (PID Tuner App)  InitialConditionSource=internal  InitialConditionForIntegrator=0  InitialConditionForFilter=0  DifferentiatorICPrevScaledInput=0  ExternalReset=none  TrackingMode=off  Kt=1  LimitOutput=on  SatLimitsSource=internal  UpperSaturationLimit=Voltage_max  LowerSaturationLimit=-Voltage_max  LinearizeAsGain=off  AntiWindupMode=none  Kb=1  LimitIntegrator=on  UpperIntegratorSaturationLimit=Voltage_max  LowerIntegratorSaturationLimit=-Voltage_max  POutMin=[]  POutMax=[]  IOutMin=[]  IOutMax=[]  DOutMin=[]  DOutMax=[]  NOutMin=[]  NOutMax=[]  SumOutMin=[]  SumOutMax=[]  SaturationOutMin=[]  SaturationOutMax=[]  PParamMin=[]  PParamMax=[]  IParamMin=[]  IParamMax=[]  DParamMin=[]  DParamMax=[]  NParamMin=[]  NParamMax=[]  KbParamMin=[]  KbParamMax=[]  KtParamMin=[]  KtParamMax=[]  KbOutMin=[]  KbOutMax=[]  KtOutMin=[]  KtOutMax=[]  IntegratorOutMin=[]  IntegratorOutMax=[]  FilterOutMin=[]  FilterOutMax=[]  SumI1OutMin=[]  SumI1OutMax=[]  SumI2OutMin=[]  SumI2OutMax=[]  SumI3OutMin=[]  SumI3OutMax=[]  SumI4OutMin=[]  SumI4OutMax=[]  SumDOutMin=[]  SumDOutMax=[]  DifferentiatorOutMin=[]  DifferentiatorOutMax=[]  FilterDiffOutCoefMin=[]  FilterDiffOutCoefMax=[]  ReciprocalOutMin=[]  ReciprocalOutMax=[]  SumDenOutMin=[]  SumDenOutMax=[]  SumNumOutMin=[]  SumNumOutMax=[]  DivideOutMin=[]  DivideOutMax=[]  UdiffTsProdOutMin=[]  UdiffTsProdOutMax=[]  NTsProdOutMin=[]  NTsProdOutMax=[]  UintegralTsProdOutMin=[]  UintegralTsProdOutMax=[]  UngainTsProdOutMin=[]  UngainTsProdOutMax=[]  ClampingZeroOutDataTypeStr=Inherit: Inherit via back propagation  ClampingZeroOutMin=[]  ClampingZeroOutMax=[]  FilterDenConstantOutDataTypeStr=Inherit: Inherit via back propagation  FilterDenConstantOutMin=[]  FilterDenConstantOutMax=[]  PCopyOutDataTypeStr=Inherit: Inherit via back propagation  PCopyOutMin=[]  PCopyOutMax=[]  NCopyOutDataTypeStr=Inherit: Inherit via back propagation  NCopyOutMin=[]  NCopyOutMax=[]  IntegratorContinuousStateAttributes=''  IntegratorStateMustResolveToSignalObject=off  IntegratorRTWStateStorageClass=Auto  FilterContinuousStateAttributes=''  FilterStateMustResolveToSignalObject=off  FilterRTWStateStorageClass=Auto  ParallelPVariant=InternalParameters  IdealPVariant=Disabled  IVariant=InternalParameters  DVariant=Disabled  IntegratorVariant=Continuous  SatVariant=Enabled  AWVariant=Passthrough  PCopyVariant=Disabled  TRVariant=Disabled  FdbkBlocksVariant=Forward  IdealPFdbkVariant=Disabled  SatFdbkVariant=Disabled  DerivativeFilterVariant=Disabled  NVariant=Disabled  NCopyVariant=Disabled_SignalSpec  FilterICVariant=Disabled  IntegratorICVariant=InternalICs  ExternalResetVariant=Disabled  TRSumVariant=Passthrough  SumFdbkVariant=Disabled  SumVariant=Sum_PI  TsampFilterVariant=InternalTs  TsampNgainVariant=Passthrough  TsampIntegralVariant=Disabled_SignalSpec  ExternalSaturationOutDataTypeStr=Inherit: Same as second input  DerivativeSourceVariant=Disabled  PreIntVariant=InternalPreInt
  I_dq PID1 : slpidlib/PID Controller  Controller=PI  Form=Parallel  TimeDomain=Continuous-time  UseExternalTs=off  SampleTime=-1  IntegratorMethod=Forward Euler  FilterMethod=Forward Euler  ControllerParametersSource=internal  P=0.199995991549269  I=7.0005743607815  UseKiTs=off  D=2.81416629288768e-05  UseExternalDerivativeSource=off  N=4271.19819316481  UseFilter=on  TunerSelectOption=Transfer Function Based (PID Tuner App)  InitialConditionSource=internal  InitialConditionForIntegrator=0  InitialConditionForFilter=0  DifferentiatorICPrevScaledInput=0  ExternalReset=none  TrackingMode=off  Kt=1  LimitOutput=on  SatLimitsSource=internal  UpperSaturationLimit=Voltage_max  LowerSaturationLimit=-Voltage_max  LinearizeAsGain=off  AntiWindupMode=none  Kb=1  LimitIntegrator=on  UpperIntegratorSaturationLimit=Voltage_max  LowerIntegratorSaturationLimit=-Voltage_max  POutMin=[]  POutMax=[]  IOutMin=[]  IOutMax=[]  DOutMin=[]  DOutMax=[]  NOutMin=[]  NOutMax=[]  SumOutMin=[]  SumOutMax=[]  SaturationOutMin=[]  SaturationOutMax=[]  PParamMin=[]  PParamMax=[]  IParamMin=[]  IParamMax=[]  DParamMin=[]  DParamMax=[]  NParamMin=[]  NParamMax=[]  KbParamMin=[]  KbParamMax=[]  KtParamMin=[]  KtParamMax=[]  KbOutMin=[]  KbOutMax=[]  KtOutMin=[]  KtOutMax=[]  IntegratorOutMin=[]  IntegratorOutMax=[]  FilterOutMin=[]  FilterOutMax=[]  SumI1OutMin=[]  SumI1OutMax=[]  SumI2OutMin=[]  SumI2OutMax=[]  SumI3OutMin=[]  SumI3OutMax=[]  SumI4OutMin=[]  SumI4OutMax=[]  SumDOutMin=[]  SumDOutMax=[]  DifferentiatorOutMin=[]  DifferentiatorOutMax=[]  FilterDiffOutCoefMin=[]  FilterDiffOutCoefMax=[]  ReciprocalOutMin=[]  ReciprocalOutMax=[]  SumDenOutMin=[]  SumDenOutMax=[]  SumNumOutMin=[]  SumNumOutMax=[]  DivideOutMin=[]  DivideOutMax=[]  UdiffTsProdOutMin=[]  UdiffTsProdOutMax=[]  NTsProdOutMin=[]  NTsProdOutMax=[]  UintegralTsProdOutMin=[]  UintegralTsProdOutMax=[]  UngainTsProdOutMin=[]  UngainTsProdOutMax=[]  ClampingZeroOutDataTypeStr=Inherit: Inherit via back propagation  ClampingZeroOutMin=[]  ClampingZeroOutMax=[]  FilterDenConstantOutDataTypeStr=Inherit: Inherit via back propagation  FilterDenConstantOutMin=[]  FilterDenConstantOutMax=[]  PCopyOutDataTypeStr=Inherit: Inherit via back propagation  PCopyOutMin=[]  PCopyOutMax=[]  NCopyOutDataTypeStr=Inherit: Inherit via back propagation  NCopyOutMin=[]  NCopyOutMax=[]  IntegratorContinuousStateAttributes=''  IntegratorStateMustResolveToSignalObject=off  IntegratorRTWStateStorageClass=Auto  FilterContinuousStateAttributes=''  FilterStateMustResolveToSignalObject=off  FilterRTWStateStorageClass=Auto  ParallelPVariant=InternalParameters  IdealPVariant=Disabled  IVariant=InternalParameters  DVariant=Disabled  IntegratorVariant=Continuous  SatVariant=Enabled  AWVariant=Passthrough  PCopyVariant=Disabled  TRVariant=Disabled  FdbkBlocksVariant=Forward  IdealPFdbkVariant=Disabled  SatFdbkVariant=Disabled  DerivativeFilterVariant=Disabled  NVariant=Disabled  NCopyVariant=Disabled_SignalSpec  FilterICVariant=Disabled  IntegratorICVariant=InternalICs  ExternalResetVariant=Disabled  TRSumVariant=Passthrough  SumFdbkVariant=Disabled  SumVariant=Sum_PI  TsampFilterVariant=InternalTs  TsampNgainVariant=Passthrough  TsampIntegralVariant=Disabled_SignalSpec  ExternalSaturationOutDataTypeStr=Inherit: Same as second input  DerivativeSourceVariant=Disabled  PreIntVariant=InternalPreInt
  Inverse park : Subsystem
  Limiter : Saturate  UpperLimit=Voltage_max  LowerLimit=0  LinearizeAsGain=off
  Limiter 1 : Saturate  UpperLimit=Voltage_max  LowerLimit=0  LinearizeAsGain=off
  Limiter1 : Saturate  UpperLimit=Current_max  LowerLimit=-Current_max  LinearizeAsGain=off
  Mux : Mux  Inputs=3
  Park Transform : spsabctodq0Lib/abc to dq0  Alignment=Aligned with phase A axis
  Saturation : Saturate  UpperLimit=speed_max  LowerLimit=-speed_max
  Scope : Scope  NumInputPorts=4
  Speed PD : slpidlib/PID Controller  Controller=PD  Form=Parallel  TimeDomain=Continuous-time  UseExternalTs=off  SampleTime=-1  IntegratorMethod=Forward Euler  FilterMethod=Forward Euler  ControllerParametersSource=internal  P=20.75762  I=640.266262711417  UseKiTs=off  D=0  UseExternalDerivativeSource=off  N=100  UseFilter=on  TunerSelectOption=Transfer Function Based (PID Tuner App)  InitialConditionSource=internal  InitialConditionForIntegrator=0  InitialConditionForFilter=0  DifferentiatorICPrevScaledInput=0  ExternalReset=none  TrackingMode=off  Kt=1  LimitOutput=on  SatLimitsSource=internal  UpperSaturationLimit=Torque_max  LowerSaturationLimit=-Torque_max  LinearizeAsGain=off  AntiWindupMode=none  Kb=1  LimitIntegrator=on  UpperIntegratorSaturationLimit=Torque_max  LowerIntegratorSaturationLimit=-Torque_max  RndMeth=Nearest  POutMin=[]  POutMax=[]  IOutMin=[]  IOutMax=[]  DOutMin=[]  DOutMax=[]  NOutMin=[]  NOutMax=[]  SumOutMin=[]  SumOutMax=[]  SaturationOutMin=[]  SaturationOutMax=[]  PParamMin=[]  PParamMax=[]  IParamMin=[]  IParamMax=[]  DParamMin=[]  DParamMax=[]  NParamMin=[]  NParamMax=[]  KbParamMin=[]  KbParamMax=[]  KtParamMin=[]  KtParamMax=[]  KbOutMin=[]  KbOutMax=[]  KtOutMin=[]  KtOutMax=[]  IntegratorOutMin=[]  IntegratorOutMax=[]  FilterOutMin=[]  FilterOutMax=[]  SumI1OutMin=[]  SumI1OutMax=[]  SumI2OutMin=[]  SumI2OutMax=[]  SumI3OutMin=[]  SumI3OutMax=[]  SumI4OutMin=[]  SumI4OutMax=[]  SumDOutMin=[]  SumDOutMax=[]  DifferentiatorOutMin=[]  DifferentiatorOutMax=[]  FilterDiffOutCoefMin=[]  FilterDiffOutCoefMax=[]  ReciprocalOutMin=[]  ReciprocalOutMax=[]  SumDenOutMin=[]  SumDenOutMax=[]  SumNumOutMin=[]  SumNumOutMax=[]  DivideOutMin=[]  DivideOutMax=[]  UdiffTsProdOutMin=[]  UdiffTsProdOutMax=[]  NTsProdOutMin=[]  NTsProdOutMax=[]  UintegralTsProdOutMin=[]  UintegralTsProdOutMax=[]  UngainTsProdOutMin=[]  UngainTsProdOutMax=[]  ClampingZeroOutDataTypeStr=Inherit: Inherit via back propagation  ClampingZeroOutMin=[]  ClampingZeroOutMax=[]  FilterDenConstantOutDataTypeStr=Inherit: Inherit via back propagation  FilterDenConstantOutMin=[]  FilterDenConstantOutMax=[]  PCopyOutDataTypeStr=Inherit: Inherit via back propagation  PCopyOutMin=[]  PCopyOutMax=[]  NCopyOutDataTypeStr=Inherit: Inherit via back propagation  NCopyOutMin=[]  NCopyOutMax=[]  IntegratorContinuousStateAttributes=''  IntegratorStateMustResolveToSignalObject=off  IntegratorRTWStateStorageClass=Auto  FilterContinuousStateAttributes=''  FilterStateMustResolveToSignalObject=off  FilterRTWStateStorageClass=Auto  ParallelPVariant=InternalParameters  IdealPVariant=Disabled  IVariant=Disabled  DVariant=InternalParameters  IntegratorVariant=Disabled  SatVariant=Enabled  AWVariant=Disabled  PCopyVariant=Disabled  TRVariant=Disabled  FdbkBlocksVariant=Forward  IdealPFdbkVariant=Disabled  SatFdbkVariant=Disabled  DerivativeFilterVariant=ContFilter  NVariant=InternalParameters  NCopyVariant=Disabled  FilterICVariant=InternalICsFilter  IntegratorICVariant=Disabled  ExternalResetVariant=Disabled  TRSumVariant=Passthrough  SumFdbkVariant=Disabled  SumVariant=Sum_PD  TsampFilterVariant=InternalTs  TsampNgainVariant=Passthrough  TsampIntegralVariant=Disabled_SignalSpec  ExternalSaturationOutDataTypeStr=Inherit: Same as second input  DerivativeSourceVariant=ErrorSignal  PreIntVariant=InternalPreInt
  Subtract : Sum  Inputs=+-
  Sum1 : Sum  Inputs=|++
  Sum3 : Sum  Inputs=|+-
  Sum4 : Sum  Inputs=|+-
  Sum6 : Sum  Inputs=|+-
  Sum7 : Sum  Inputs=|++
  Switch : Switch  Criteria=u2 > Threshold  SaturateOnIntegerOverflow=off  InputSameDT=off
  Terminator : Terminator
  Out1 : Outport
  Out2 : Outport  Port=2
  Out3 : Outport  Port=3
  Out4 : Outport  Port=4
  Out5 : Outport  Port=5
  wires:
  In5/1 -> Mux/2  "Ib"
  In6/1 -> Mux/3  "Ic"
  Derivative/1 -> Sum6/2, Decoupling/3(Speed)  "Electrical speed (Rad/s)"
  I_dq PID1/1 -> Sum1/1
  [Id] -> Scope/2, Sum4/2
  Demux/2 -> [Iq]  "Iq"
  Inverse park/1(Duty Cycle A) -> Out1/1  "Va*"
  I_dq PID/1 -> Sum7/1
  Inverse park/3(Duty Cycle A2) -> Out3/1  "Vc*"
  [Iq] -> Scope/1, Sum3/2
  Switch/1 -> Scope/4, Out4/1, Gain6/1  "Te*"
  Demux/1 -> [Id]  "Id"
  [Iq] -> Decoupling/1(Iq)
  Demux/3 -> Terminator/1
  Sum3/1 -> I_dq PID/1  "Iq_error"
  Decoupling/2(Eq) -> Sum1/2  "Ed"
  Sum7/1 -> Limiter/1
  Limiter 1/1 -> Inverse park/2(Iq)  "Vd*"
  Decoupling/1(Ed) -> Sum7/2  "Eq"
  In1/1 -> Saturation/1  "User_Spd_Req"
  Inverse park/2(Duty Cycle A1) -> Out2/1  "Vb*"
  Sum4/1 -> I_dq PID1/1  "Id_err"
  Sum1/1 -> Limiter 1/1
  Sum6/1 -> Speed PD/1  "speed_err"
  Constant1/1 -> Sum4/1  "id*"
  Speed PD/1 -> Switch/3  "PID_Torque Req"
  [Id] -> Decoupling/2(Id)
  In4/1 -> Mux/1  "Ia"
  Limiter/1 -> Inverse park/1(Vq)  "Vq*"
  Mux/1 -> Park Transform/1
  Gain6/1 -> Limiter1/1
  In3/1 -> Switch/1  "User_Tourqe_Req"
  Park Transform/1 -> Demux/1
  In2/1 -> Subtract/1  "Rotor Angle"
  In7/1 -> Switch/2  "Speed/!Torque mode"
  Limiter1/1 -> Scope/3, Sum3/1  "Iq*"
  Gain7/1 -> Sum6/1  "We*"
  Gain2/1 -> Derivative/1, Park Transform/2, Inverse park/3(In3)  "Electrical speed"
  Const/1 -> Subtract/2
  Subtract/1 -> Gain2/1
  Saturation/1 -> Out5/1, Gain7/1

== system Minh_Final_project_Inverter_V3/Ideal Simulation Continous Time/PMSM Mathematical model ==
  note: PMSM (Mathematical Model)
  abc : Inport
  Constant : Constant  Value=Encoder_Offset
  Constant3 : Constant  Value=0
  Demux1 : Demux  Outputs=3
  Gain6 : Gain  Gain=1/ppair
  Machine Model in DQ : Subsystem
  Mechanical Model : Subsystem
  Mux1 : Mux  Inputs=3
  Sum : Sum  Inputs=|++
  Terminator : Terminator
  abc to dq0 : spsabctodq0Lib/abc to dq0  Alignment=Aligned with phase A axis
  dq0 to abc : spsdq0toabcLib/dq0 to abc  Alignment=Aligned with phase A axis
  abc1 : Outport
  Out3 : Outport  Port=2
  T_e : Outport  Port=3
  w_m : Outport  Port=4
  wires:
  Demux1/2 -> Machine Model in DQ/2(v_q)
  Machine Model in DQ/3(th_e) -> abc to dq0/2, dq0 to abc/2, Gain6/1
  Demux1/1 -> Machine Model in DQ/1(v_d)
  Mux1/1 -> dq0 to abc/1
  Mechanical Model/1(w_m) -> w_m/1, Machine Model in DQ/3(w_m)
  Machine Model in DQ/4(T_e) -> T_e/1, Mechanical Model/1(T_e)  "Tourqe"
  Constant3/1 -> Mux1/3
  Demux1/3 -> Terminator/1
  Machine Model in DQ/1(i_d) -> Mux1/1  "i_d"
  Machine Model in DQ/2(i_q) -> Mux1/2  "i_q"
  abc to dq0/1 -> Demux1/1
  dq0 to abc/1 -> abc1/1
  abc/1 -> abc to dq0/1
  Gain6/1 -> Sum/1  "Rotor Angle"
  Constant/1 -> Sum/2
  Sum/1 -> Out3/1  "Rotor Angle"
